simulink model "Motor_control_simulation"  (R2018a)
settings: Solver=VariableStepAuto  StartTime=0.0  StopTime=20  RelTol=1e-3
values from neighbouring files (symbols this model uses):
  turn = 45    [motor_control_simulation.m]
undefined symbols (not defined in the file or in its folder): DiscIntNeverNeededParam
settings Model: Creator=Hannes  LastModifiedBy=Hannes

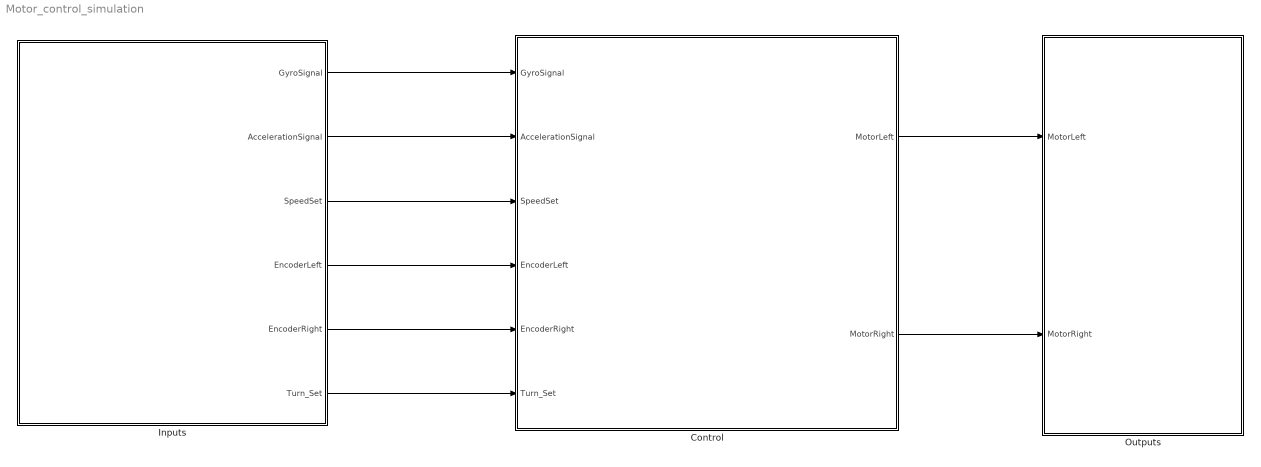
== system Motor_control_simulation ==
  Control : Subsystem
  Inputs : Subsystem
  "Outputs " : Subsystem
  wires:
  Inputs/1(GyroSignal) -> Control/1(GyroSignal)
  Inputs/6(Turn_Set) -> Control/6(Turn_Set)
  Inputs/2(AccelerationSignal) -> Control/2(AccelerationSignal)
  Inputs/3(SpeedSet) -> Control/3(SpeedSet)
  Inputs/4(EncoderLeft) -> Control/4(EncoderLeft)
  Inputs/5(EncoderRight) -> Control/5(EncoderRight)
  Control/1(MotorLeft) -> "Outputs "/1(MotorLeft)
  Control/2(MotorRight) -> "Outputs "/2(MotorRight)

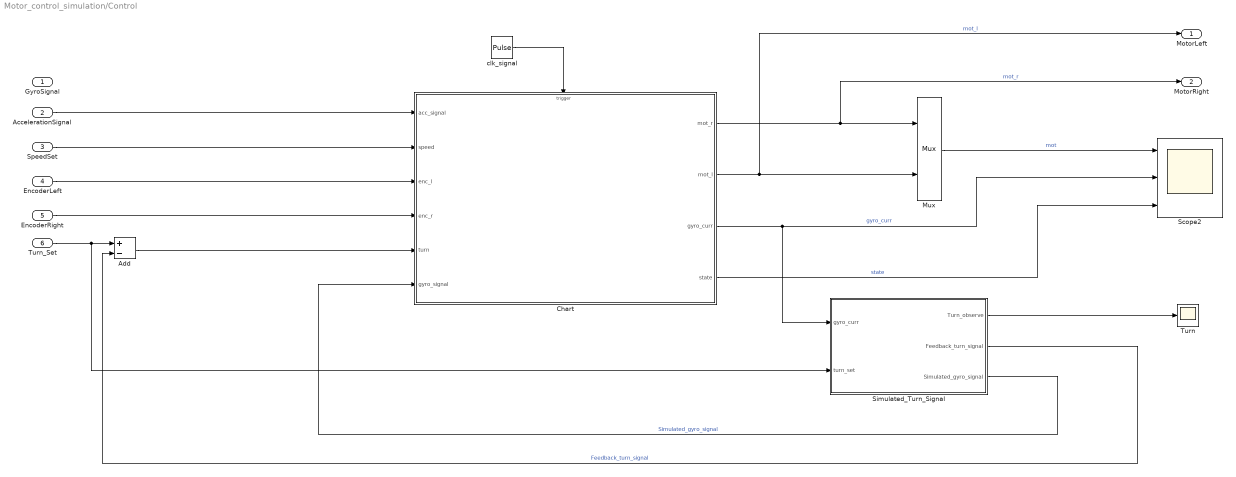
== system Motor_control_simulation/Control ==
  GyroSignal : Inport
  AccelerationSignal : Inport  Port=2
  SpeedSet : Inport  Port=3
  EncoderLeft : Inport  Port=4
  EncoderRight : Inport  Port=5
  Turn_Set : Inport  Port=6
  Add : Sum  Inputs=+-
  Chart : Stateflow chart  TreatAsAtomicUnit=on
  Mux : Mux  Inputs=2
  Scope2 : Scope  NumInputPorts=3
  Simulated_Turn_Signal : Subsystem
  Turn : Scope
  clk_signal : DiscretePulseGenerator  SampleTime=0.1
  MotorLeft : Outport
  MotorRight : Outport  Port=2
  wires:
  SpeedSet/1 -> Chart/2(speed)
  EncoderLeft/1 -> Chart/3(enc_l)
  EncoderRight/1 -> Chart/4(enc_r)
  AccelerationSignal/1 -> Chart/1(acc_signal)
  clk_signal/1 -> Chart/Trigger
  Chart/1(mot_r) -> MotorRight/1, Mux/1  "mot_r"
  Chart/2(mot_l) -> Mux/2, MotorLeft/1  "mot_l"
  Chart/3(gyro_curr) -> Simulated_Turn_Signal/1(gyro_curr), Scope2/2  "gyro_curr"
  Chart/4(state) -> Scope2/3  "state"
  Mux/1 -> Scope2/1  "mot"
  Simulated_Turn_Signal/3(Simulated_gyro_signal) -> Chart/6(gyro_signal)  "Simulated_gyro_signal"
  Simulated_Turn_Signal/1(Turn_observe) -> Turn/1
  Turn_Set/1 -> Simulated_Turn_Signal/2(turn_set), Add/1
  Simulated_Turn_Signal/2(Feedback_turn_signal) -> Add/2  "Feedback_turn_signal"
  Add/1 -> Chart/5(turn)

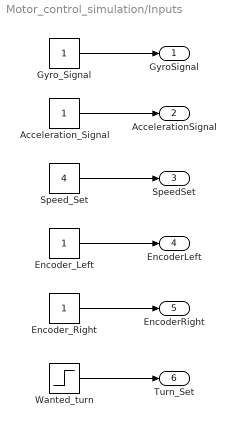
== system Motor_control_simulation/Inputs ==
  Acceleration_Signal : Constant
  Encoder_Left : Constant
  Encoder_Right : Constant
  Gyro_Signal : Constant
  Speed_Set : Constant  Value=4
  Wanted_turn : Step  Time=3  After=turn  SampleTime=0
  GyroSignal : Outport
  AccelerationSignal : Outport  Port=2
  SpeedSet : Outport  Port=3
  EncoderLeft : Outport  Port=4
  EncoderRight : Outport  Port=5
  Turn_Set : Outport  Port=6
  wires:
  Speed_Set/1 -> SpeedSet/1
  Encoder_Left/1 -> EncoderLeft/1
  Acceleration_Signal/1 -> AccelerationSignal/1
  Encoder_Right/1 -> EncoderRight/1
  Wanted_turn/1 -> Turn_Set/1
  Gyro_Signal/1 -> GyroSignal/1

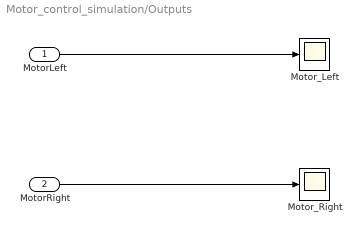
== system Motor_control_simulation/Outputs  ==
  MotorLeft : Inport
  MotorRight : Inport  Port=2
  Motor_Left : Scope
  Motor_Right : Scope
  wires:
  MotorLeft/1 -> Motor_Left/1
  MotorRight/1 -> Motor_Right/1

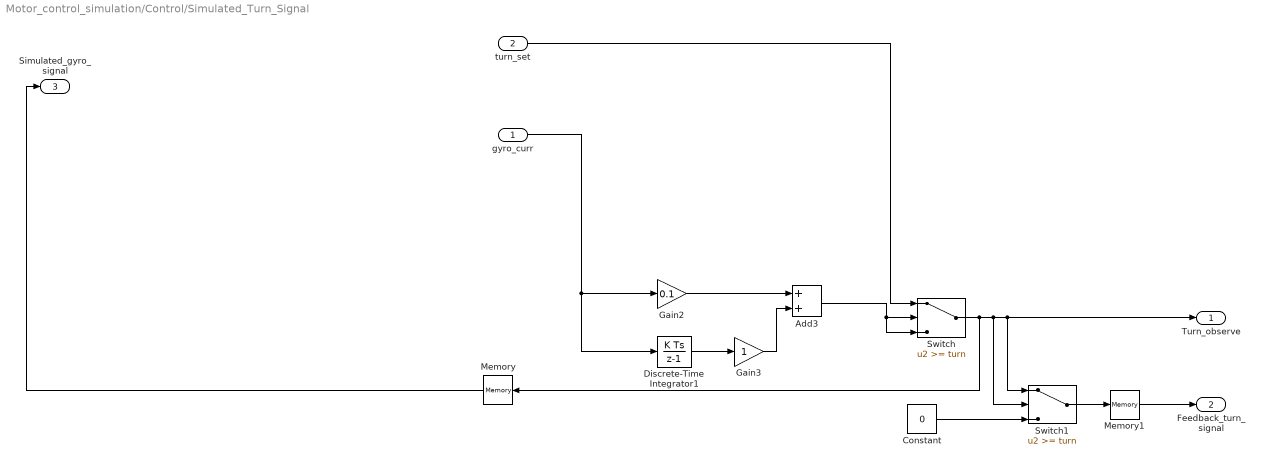
== system Motor_control_simulation/Control/Simulated_Turn_Signal ==
  gyro_curr : Inport
  turn_set : Inport  Port=2
  Add3 : Sum
  Constant : Constant  Value=0
  Discrete-Time Integrator1 : DiscreteIntegrator  gainval=0.1  SampleTime=0.5  ICPrevOutput=DiscIntNeverNeededParam  ICPrevScaledInput=DiscIntNeverNeededParam
  Gain2 : Gain  Gain=0.1
  Gain3 : Gain
  Memory : Memory  InheritSampleTime=on
  Memory1 : Memory  InheritSampleTime=on
  Switch : Switch  Threshold=turn
  Switch1 : Switch  Threshold=turn
  Turn_observe : Outport
  Feedback_turn_signal : Outport  Port=2
  Simulated_gyro_signal : Outport  Port=3
  wires:
  Gain2/1 -> Add3/1
  Discrete-Time Integrator1/1 -> Gain3/1
  gyro_curr/1 -> Discrete-Time Integrator1/1, Gain2/1
  Memory/1 -> Simulated_gyro_signal/1
  Gain3/1 -> Add3/2
  Switch/1 -> Memory/1, Switch1/2, Switch1/1, Turn_observe/1
  Add3/1 -> Switch/3, Switch/2
  turn_set/1 -> Switch/1
  Constant/1 -> Switch1/3
  Switch1/1 -> Memory1/1
  Memory1/1 -> Feedback_turn_signal/1

== stateflow chart Motor_control_simulation/Control/Chart ==
  settings: executeAtInitialization=1
  state Turn_Left
    entry: mot_l=-speed; mot_r=speed;
    gyro_curr=turn; state=5;
    during: mot_l=-speed; mot_r=speed;
    gyro_curr=turn;
    exit: mot_l=0; mot_r=0;
  state Turn_Right
    entry: mot_l=speed; mot_r=-speed;
    gyro_curr=turn; state=4;
    during: mot_l=speed; mot_r=-speed;
    gyro_curr=turn;
    exit: mot_l=0; mot_r=0;
  state Idle
    entry:mot_l=0; mot_r=0; state=1;
    during:mot_l=0; mot_r=0;
  state Backward
    entry: mot_l=speed; mot_r=speed; state=2
    during: mot_l=speed; mot_r=speed;
    exit: mot_l=0; mot_r=0;
  state Forward
    entry: mot_l=speed; mot_r=speed; state=3;
    during: mot_l=speed; mot_r=speed;
    exit: mot_l=0; mot_r=0;
  Turn_Left -> Idle : ev_clk[gyro_signal>=gyro_curr]{curr_angle=0}
  Idle -> Turn_Left [order 3] : ev_clk[turn>0]{curr_angle=gyro_signal; gyro_curr=0;}
  Idle -> Turn_Right [order 1] : ev_clk[turn<0]{curr_angle=gyro_signal; gyro_curr=0;}
  Idle -> Backward [order 2] : ev_clk[speed<0]
  Backward -> Idle : ev_clk[speed>=0 || turn ~=0 ]
  Turn_Right -> Idle : ev_clk[gyro_signal<=turn]{curr_angle=0;}
  Idle -> Forward [order 4] : ev_clk[speed>0]
  Forward -> Idle : ev_clk[speed<=0 || turn ~= 0]
  (default) -> Idle
  data: curr_angle local; acc_signal input; speed input; enc_l input; enc_r input; turn input; mot_r output; mot_l output; gyro_signal input; gyro_curr output; state output
  events: ev_clk input RISING_EDGE_EVENT
